simulink model "ASM_Traffic_V2X_Complete_Model_2"  (R2019a)
settings: Solver=ode1  StartTime=SIM.tstart.v  StopTime=Inf  FixedStep=SIM.StepSize.v  RelTol=1e-3
PostLoadFcn:
  | if any(exist('dsrtsu_mdlpostloadfcn', 'file') ~= 0), dsrtsu_mdlpostloadfcn('Execute', bdroot); end
  | try, asm_mdl_postloadfcn(bdroot, 'UpdateModel', 2200); catch, disp(lasterr); end,
undefined symbols (not defined in the file): _SensorPnts_1, _SensorPnts_13, _SensorPnts_17, _SensorPnts_21, _SensorPnts_25, _SensorPnts_29, _SensorPnts_33, _SensorPnts_37, _SensorPnts_41, _SensorPnts_45, _SensorPnts_49, _SensorPnts_5, _SensorPnts_53, _SensorPnts_57, _SensorPnts_9, _to_, CPT, G5A, ITS, MDL, rad, s_to_rpm, SIM
libraries: simulink x169, ASM_VehicleDynamics_lib x126, ASM_Traffic_lib x83, ASM_Utils_lib x49, mdbs x45, ASM_Environment_lib x17, dspindex x12, dsaV2xLibraryAux x10, dsmpblib x6, dsaV2xAsn1Library x4, dsaV2xLibrary x4, ASM_BrakeHydraulics_lib x4
(part 19 of 36)

== system ASM_Traffic_V2X_Complete_Model_2/MDL/Drivetrain/Transmission/AutomaticTransmission/ASMSignalCollector ==
  BusCreator : BusCreator  Inputs=3
  Signal Conversion : SignalConversion  OverrideOpt=off
  ASMSignalBus : Outport
  wires:
  [ASMBUS_Drivetrain_AutomaticTransmission_TorqueConverter] -> BusCreator/3
  BusCreator/1 -> Signal Conversion/1
  [ASMBUS_Drivetrain_AutomaticTransmission_Gearbox] -> BusCreator/2
  [ASMBUS_Drivetrain_AutomaticTransmission_LockUpClutch] -> BusCreator/1
  Signal Conversion/1 -> ASMSignalBus/1  "AutomaticTransmission"

== system ASM_Traffic_V2X_Complete_Model_2/MDL/Drivetrain/Transmission/AutomaticTransmission/Torque_Summation ==
  Trq_Fric[Nm] : Inport
  Trq_Out_LockupClutch[Nm] : Inport  Port=2
  Trq_Pump[Nm] : Inport  Port=3
  Trq_Turbine[Nm] : Inport  Port=4
  Sum1 : Sum  Inputs=2  SaturateOnIntegerOverflow=on  InputSameDT=on  OutDataTypeStr=Inherit: Same as first input
  Sum5 : Sum  Inputs=2  SaturateOnIntegerOverflow=on  InputSameDT=on  OutDataTypeStr=Inherit: Same as first input
  Trq_In_Converter[Nm] : Outport  InitialOutput=0
  Trq_In_Trm[Nm] : Outport  Port=2
  wires:
  Trq_Pump[Nm]/1 -> Sum5/1
  Sum1/1 -> Trq_In_Trm[Nm]/1
  Sum5/1 -> Trq_In_Converter[Nm]/1
  Trq_Fric[Nm]/1 -> Sum5/2
  Trq_Out_LockupClutch[Nm]/1 -> Sum1/1
  Trq_Turbine[Nm]/1 -> Sum1/2

== system ASM_Traffic_V2X_Complete_Model_2/MDL/Drivetrain/Transmission/ManualTransmission/ASMSignalCollector ==
  BusCreator : BusCreator  Inputs=2
  Signal Conversion : SignalConversion  OverrideOpt=off
  ASMSignalBus : Outport
  wires:
  BusCreator/1 -> Signal Conversion/1
  [ASMBUS_Drivetrain_ManualTransmission_Gearbox] -> BusCreator/2
  [ASMBUS_Drivetrain_ManualTransmission_Clutch] -> BusCreator/1
  Signal Conversion/1 -> ASMSignalBus/1  "ManualTransmission"

== system ASM_Traffic_V2X_Complete_Model_2/MDL/Environment/Driver/LateralController/ASMSignalCollector ==
  s_Preview_LatCtrl[m] : Inport
  Angle_SteeringWheel_LatCtrl[deg] : Inport  Port=2
  e_Lat[m] : Inport  Port=3
  Bus Creator : BusCreator  Inputs=3
  Bus Creator1 : BusCreator  Inputs=4
  Max : MinMax  Function=max  SaturateOnIntegerOverflow=on  InputSameDT=on
  tag scope: ASMBUS_Env_Driver_LatController=global
  wires:
  [ASMBUS_Env_Driver_LatCtrl_PosError] -> Bus Creator1/4
  Max/1 -> Bus Creator/1  "s_Preview_LatCtrl[m]"
  Angle_SteeringWheel_LatCtrl[deg]/1 -> Bus Creator/2  "Angle_SteeringWheel_LatCtrl[deg]"
  Bus Creator1/1 -> [ASMBUS_Env_Driver_LatController]  "LateralController"
  [ASMBUS_Env_Driver_LatCtrl2] -> Bus Creator1/3
  [ASMBUS_Env_Driver_LatCtrl1] -> Bus Creator1/2
  Bus Creator/1 -> Bus Creator1/1  "ActiveLateralController"
  e_Lat[m]/1 -> Bus Creator/3  "e_Lat[m]"
  s_Preview_LatCtrl[m]/1 -> Max/1  "s_Preview_LatCtrl[m]"

== system ASM_Traffic_V2X_Complete_Model_2/MDL/Environment/Driver/LongitudinalController/ASMSignalCollector ==
  Bus Creator : BusCreator  Inputs=2
  tag scope: ASMBUS_Env_Driver_LongController=global
  wires:
  [ASMBUS_Env_Driver_GearShifter] -> Bus Creator/2
  [ASMBUS_Env_Driver_LongCtrl] -> Bus Creator/1
  Bus Creator/1 -> [ASMBUS_Env_Driver_LongController]  "LongitudinalController"

== system ASM_Traffic_V2X_Complete_Model_2/MDL/Environment/Driver/LongitudinalController/Default_GearClutch_Mode ==
  note: For automatic transmission, the default value of GearClutch_Mode is set to the Driver Mode
  GearClutch_Mode[1Stim|2Driver|3OpenClutch|4RefGear] : Inport
  Automatic_Transmission : simulink/Logic and Bit Operations/Compare To Constant  relop===  const=2  OutDataTypeStr=boolean
  GearClutch_Mode[2Driver] : Constant  Value=2
  Multiport Switch : MultiPortSwitch  Inputs=2
  Sw_GearClutchMode[1Driver|2Others] : Constant
  Switch : Switch  Criteria=u2 ~= 0
  GearClutch_Mode[1Stim|2Driver|3OpenClutch|4RefGear]_ : Outport  OutputWhenDisabled=reset  InitialOutput=0
  wires:
  Multiport Switch/1 -> Switch/1
  Sw_GearClutchMode[1Driver|2Others]/1 -> Multiport Switch/1
  GearClutch_Mode[2Driver]/1 -> Multiport Switch/2
  GearClutch_Mode[1Stim|2Driver|3OpenClutch|4RefGear]/1 -> Multiport Switch/3, Switch/3
  Switch/1 -> GearClutch_Mode[1Stim|2Driver|3OpenClutch|4RefGear]_/1
  Automatic_Transmission/1 -> Switch/2
  [TAG_Sw_Transmission_Mode] -> Automatic_Transmission/1

== system ASM_Traffic_V2X_Complete_Model_2/MDL/Environment/Driver/LongitudinalController/Driving_Resistances ==
  VehicleDynamics_Signals : Inport
  Add : Sum  Inputs=+++
  Bus Selector1 : BusSelector  OutputSignals=VehicleMovement.Forces.F_x_Vehicle_Gravitational[N],VehicleMovement.Forces.F_x_Aero_CoorSys_V[N],VehicleMovement.Forces.F_z_Vehicle_Gravitational[N],Tire.Coef_RollingRes_Mean[]
  Gain : Gain  Gain=-1
  Gain1 : Gain
  Gain2 : Gain
  Product2 : Product  RndMeth=Zero
  F_Tractive_Res[N] : Outport
  wires:
  Gain1/1 -> Add/2  "F_Slope[N]"
  Gain2/1 -> Add/1  "F_Aerodynamics[N]"
  Bus Selector1/3 -> Product2/1  "<F_z_Vehicle_Gravitational[N]>"
  Bus Selector1/2 -> Gain1/1  "<F_x_Aero_CoorSys_V[N]>"
  Bus Selector1/1 -> Gain2/1  "<F_x_Vehicle_Gravitational[N]>"
  Gain/1 -> F_Tractive_Res[N]/1
  Add/1 -> Gain/1  "Driving_Res[N]"
  Product2/1 -> Add/3  "F_Roll[N]"
  Bus Selector1/4 -> Product2/2  "<Coef_RollingRes_Mean[]>"
  VehicleDynamics_Signals/1 -> Bus Selector1/1

== system ASM_Traffic_V2X_Complete_Model_2/MDL/Environment/Driver/ReferenceVelocity/Extend_Dimension ==
  In : Inport
  Selector : Selector  InputPortWidth=10  IndexOptions=Index vector (dialog)  Indices=[1:10,10,10,10,10,10]  OutputSizes=1
      settings: AttributesFormatString=|
      | PortWidth = %<InputPortWidth>
      | Indices = %<Indices>
  Out : Outport
  wires:
  In/1 -> Selector/1
  Selector/1 -> Out/1

== system ASM_Traffic_V2X_Complete_Model_2/MDL/Environment/Driver/ReferenceVelocity/Reduce_Dimension2 ==
  In : Inport
  Selector : Selector  InputPortWidth=15  IndexOptions=Index vector (dialog)  Indices=[1:10]  OutputSizes=1
      settings: AttributesFormatString=|
      | PortWidth = %<InputPortWidth>
      | Indices = %<Indices>
  Out : Outport
  wires:
  Selector/1 -> Out/1
  In/1 -> Selector/1

== system ASM_Traffic_V2X_Complete_Model_2/MDL/Environment/Driver/ReferenceVelocity/Reduce_Dimension3 ==
  In : Inport
  Selector : Selector  InputPortWidth=15  IndexOptions=Index vector (dialog)  Indices=[1:10]  OutputSizes=1
      settings: AttributesFormatString=|
      | PortWidth = %<InputPortWidth>
      | Indices = %<Indices>
  Out : Outport
  wires:
  In/1 -> Selector/1
  Selector/1 -> Out/1

== system ASM_Traffic_V2X_Complete_Model_2/MDL/Environment/Driver/ReferenceVelocity/Reduce_Dimension4 ==
  In : Inport
  Selector : Selector  InputPortWidth=15  IndexOptions=Index vector (dialog)  Indices=[1:10]  OutputSizes=1
      settings: AttributesFormatString=|
      | PortWidth = %<InputPortWidth>
      | Indices = %<Indices>
  Out : Outport
  wires:
  Selector/1 -> Out/1
  In/1 -> Selector/1

== system ASM_Traffic_V2X_Complete_Model_2/MDL/Environment/Driver/ReferenceVelocity/Reduce_Dimension5 ==
  In : Inport
  Selector : Selector  InputPortWidth=15  IndexOptions=Index vector (dialog)  Indices=[1:10]  OutputSizes=1
      settings: AttributesFormatString=|
      | PortWidth = %<InputPortWidth>
      | Indices = %<Indices>
  Out : Outport
  wires:
  Selector/1 -> Out/1
  In/1 -> Selector/1

== system ASM_Traffic_V2X_Complete_Model_2/MDL/Environment/Driver/SignalSelection/ASMSignalCollector ==
  Driver_Signals : Inport
  tag scope: ASMBUS_Env_Driver_SignalSelection=global
  wires:
  Driver_Signals/1 -> [ASMBUS_Env_Driver_SignalSelection]  "OutputSignals"

== system ASM_Traffic_V2X_Complete_Model_2/MDL/Environment/Driver/Source_of_eGoCAR_Control_Conditions/Steer_Decision_Conditions ==
  In1 : Inport
  AND : Logic  IconShape=distinctive  AllPortsSameDT=off  OutDataTypeStr=boolean
  Clock : Clock
  Data Type Conversion : DataTypeConversion  OutDataTypeStr=double
  Min_Speed_for_Manueveur : Constant  Value=50
  Min_Time_for_Manueveur : Constant  Value=10
  Relational Operator : RelationalOperator  OutDataTypeStr=boolean  RndMeth=Simplest
  Relational Operator1 : RelationalOperator  Operator=<=  OutDataTypeStr=boolean  RndMeth=Simplest
  Out1 : Outport
  wires:
  Relational Operator1/1 -> AND/2
  AND/1 -> Data Type Conversion/1
  Relational Operator/1 -> AND/1
  Min_Speed_for_Manueveur/1 -> Relational Operator1/2
  In1/1 -> Relational Operator1/1
  Clock/1 -> Relational Operator/1
  Min_Time_for_Manueveur/1 -> Relational Operator/2
  Data Type Conversion/1 -> Out1/1

== system ASM_Traffic_V2X_Complete_Model_2/MDL/Environment/EnvironmentInterface_In/Drivetrain/Mapping ==
  n_Engine[rpm]_ : Inport
  omega_Out_Trm[rad|s]_ : Inport  Port=2
  Bus Creator : BusCreator  Inputs=2
  n_Engine[rpm] : Subsystem
      mask Display: disp('')
  omega_Out_Trm[rad|s] : Subsystem
      mask Display: disp('')
  Out : Outport
  wires:
  omega_Out_Trm[rad|s]/1(Out1) -> Bus Creator/2  "omega_Out_Trm[rad|s]"
  n_Engine[rpm]/1(Out1) -> Bus Creator/1  "n_Engine[rpm]"
  omega_Out_Trm[rad|s]_/1 -> omega_Out_Trm[rad|s]/1(In1)
  n_Engine[rpm]_/1 -> n_Engine[rpm]/1(In1)
  Bus Creator/1 -> Out/1  "Drivetrain"

== system ASM_Traffic_V2X_Complete_Model_2/MDL/Environment/EnvironmentInterface_In/SoftECU_Engine/Mapping ==
  Const_n_Engine_Idle_Set[rpm] : Inport
  State_Engine[0|1|2|3|4] : Inport  Port=2
  FCW[0Off|1On] : Inport  Port=3
  AEB[0Off|1On] : Inport  Port=4
  AEB[0Off|1On]1 : Subsystem
      mask Display: disp('')
  Bus Creator : BusCreator  Inputs=2
  Bus Creator1 : BusCreator  Inputs=2
  Bus Creator2 : BusCreator  Inputs=2
  Const_n_Engine_Idle_Set[rpm]1 : Subsystem
      mask Display: disp('')
  FCW[0Off|1On]1 : Subsystem
      mask Display: disp('')
  State_Engine[0|1|2|3|4]_ : Subsystem
      mask Display: disp('')
  Out : Outport
  wires:
  State_Engine[0|1|2|3|4]_/1(Out1) -> Bus Creator/2  "State_Engine[0|1|2|3|4]"
  State_Engine[0|1|2|3|4]/1 -> State_Engine[0|1|2|3|4]_/1(In1)
  Bus Creator2/1 -> Out/1  "SoftECU"
  Bus Creator1/1 -> Bus Creator2/2  "SoftECU_ACC"
  Bus Creator/1 -> Bus Creator2/1  "SoftECU_Engine"
  AEB[0Off|1On]1/1(Out1) -> Bus Creator1/2  "AEB[0Off|1On]"
  FCW[0Off|1On]1/1(Out1) -> Bus Creator1/1  "FCW[0Off|1On]"
  AEB[0Off|1On]/1 -> AEB[0Off|1On]1/1(In1)
  FCW[0Off|1On]/1 -> FCW[0Off|1On]1/1(In1)
  Const_n_Engine_Idle_Set[rpm]1/1(Out1) -> Bus Creator/1  "Const_n_Engine_Idle_Set[rpm]"
  Const_n_Engine_Idle_Set[rpm]/1 -> Const_n_Engine_Idle_Set[rpm]1/1(In1)

== system ASM_Traffic_V2X_Complete_Model_2/MDL/Environment/EnvironmentInterface_In/Steering/Mapping ==
  i_Steering_Mean[] : Inport
  Angle_SteeringWheel[deg] : Inport  Port=2
  Trq_SteeringWheel[Nm] : Inport  Port=3
  Angle_SteeringWheel[deg]1 : Subsystem
      mask Display: disp('')
  Bus Creator : BusCreator  Inputs=3
  Trq_SteeringWheel[Nm]1 : Subsystem
      mask Display: disp('')
  i_Steering_Mean[]1 : Subsystem
      mask Display: disp('')
  Out : Outport
  wires:
  Angle_SteeringWheel[deg]1/1(Out1) -> Bus Creator/2  "Angle_SteeringWheel[deg]"
  Trq_SteeringWheel[Nm]1/1(Out1) -> Bus Creator/3  "Trq_SteeringWheel[Nm]"
  Angle_SteeringWheel[deg]/1 -> Angle_SteeringWheel[deg]1/1(In1)
  Trq_SteeringWheel[Nm]/1 -> Trq_SteeringWheel[Nm]1/1(In1)
  i_Steering_Mean[]/1 -> i_Steering_Mean[]1/1(In1)
  i_Steering_Mean[]1/1(Out1) -> Bus Creator/1  "i_Steering_Mean[]"
  Bus Creator/1 -> Out/1  "Steering"

== system ASM_Traffic_V2X_Complete_Model_2/MDL/Environment/EnvironmentInterface_In/Tire/Mapping ==
  r_Dyn_Tire_Mean[m] : Inport
  Coef_RollingRes_Mean[] : Inport  Port=2
  CorneringStiffness_Tire_Front[N|rad] : Inport  Port=3
  CorneringStiffness_Tire_Rear[N|rad] : Inport  Port=4
  Pos_CP_FL_CoorSys_E[x;y][m] : Inport  Port=5
  Pos_CP_FR_CoorSys_E[x;y][m] : Inport  Port=6
  Pos_CP_RL_CoorSys_E[x;y][m] : Inport  Port=7
  Pos_CP_RR_CoorSys_E[x;y][m] : Inport  Port=8
  Bus Creator : BusCreator  Inputs=5
  Coef_RollingRes_Mean[]1 : Subsystem
      mask Display: disp('')
  CorneringStiffness_Tire_Front[N|rad]1 : Subsystem
      mask Display: disp('')
  CorneringStiffness_Tire_Rear[N|rad]1 : Subsystem
      mask Display: disp('')
  Mux : Mux
  r_Dyn_Tire_Mean[m]1 : Subsystem
      mask Display: disp('')
  Out : Outport
  wires:
  Mux/1 -> Bus Creator/5  "Pos_CP_CoorSys_E[:][x;y][m]"
  CorneringStiffness_Tire_Rear[N|rad]/1 -> CorneringStiffness_Tire_Rear[N|rad]1/1(In1)
  CorneringStiffness_Tire_Front[N|rad]/1 -> CorneringStiffness_Tire_Front[N|rad]1/1(In1)
  Coef_RollingRes_Mean[]/1 -> Coef_RollingRes_Mean[]1/1(In1)
  r_Dyn_Tire_Mean[m]/1 -> r_Dyn_Tire_Mean[m]1/1(In1)
  CorneringStiffness_Tire_Rear[N|rad]1/1(Out1) -> Bus Creator/4  "CorneringStiffness_Tire_Rear[N|rad]"
  CorneringStiffness_Tire_Front[N|rad]1/1(Out1) -> Bus Creator/3  "CorneringStiffness_Tire_Front[N|rad]"
  Coef_RollingRes_Mean[]1/1(Out1) -> Bus Creator/2  "Coef_RollingRes_Mean[]"
  r_Dyn_Tire_Mean[m]1/1(Out1) -> Bus Creator/1  "r_Dyn_Tire_Mean[m]"
  Pos_CP_RR_CoorSys_E[x;y][m]/1 -> Mux/4
  Pos_CP_RL_CoorSys_E[x;y][m]/1 -> Mux/3
  Pos_CP_FR_CoorSys_E[x;y][m]/1 -> Mux/2
  Pos_CP_FL_CoorSys_E[x;y][m]/1 -> Mux/1
  Bus Creator/1 -> Out/1  "Tire"

== system ASM_Traffic_V2X_Complete_Model_2/MDL/Environment/EnvironmentInterface_In/VehicleMovement/Mapping ==
  m_TotalVehicle[kg] : Inport
  Pos_x_CoG_Vehicle_Total[m] : Inport  Port=2
  Inertia_z_Vehicle_Total[kgm2] : Inport  Port=3
  Bus Creator : BusCreator  Inputs=3
  Inertia_z_Vehicle_Total[kgm2]1 : Subsystem
      mask Display: disp('')
  Pos_x_CoG_Vehicle_Total[m]1 : Subsystem
      mask Display: disp('')
  m_TotalVehicle[kg]1 : Subsystem
      mask Display: disp('')
  Out : Outport
  wires:
  Bus Creator/1 -> Out/1  "Parameters"
  m_TotalVehicle[kg]1/1(Out1) -> Bus Creator/1  "m_TotalVehicle[kg]"
  Pos_x_CoG_Vehicle_Total[m]1/1(Out1) -> Bus Creator/2  "Pos_x_CoG_Vehicle_Total[m]"
  Inertia_z_Vehicle_Total[kgm2]1/1(Out1) -> Bus Creator/3  "Inertia_z_Vehicle_Total[kgm2]"
  m_TotalVehicle[kg]/1 -> m_TotalVehicle[kg]1/1(In1)
  Pos_x_CoG_Vehicle_Total[m]/1 -> Pos_x_CoG_Vehicle_Total[m]1/1(In1)
  Inertia_z_Vehicle_Total[kgm2]/1 -> Inertia_z_Vehicle_Total[kgm2]1/1(In1)

== system ASM_Traffic_V2X_Complete_Model_2/MDL/Environment/EnvironmentInterface_In/VehicleMovement/Mapping_Acc ==
  a_y_Vehicle_CoG[m|s2] : Inport
  Bus Creator : BusCreator  Inputs=1
  a_y_Vehicle_CoG[m|s2]1 : Subsystem
      mask Display: disp('')
  Out : Outport
  wires:
  Bus Creator/1 -> Out/1  "Accelerations"
  a_y_Vehicle_CoG[m|s2]1/1(Out1) -> Bus Creator/1  "a_y_Vehicle_CoG[m|s2]"
  a_y_Vehicle_CoG[m|s2]/1 -> a_y_Vehicle_CoG[m|s2]1/1(In1)

== system ASM_Traffic_V2X_Complete_Model_2/MDL/Environment/EnvironmentInterface_In/VehicleMovement/Mapping_F ==
  F_x_Vehicle_Gravitational[N] : Inport
  F_z_Vehicle_Gravitational[N] : Inport  Port=2
  F_x_Aero_CoorSys_V[N] : Inport  Port=3
  Bus Creator : BusCreator  Inputs=3
  F_x_Aero_CoorSys_V[N]1 : Subsystem
      mask Display: disp('')
  F_x_Vehicle_Gravitational[N]1 : Subsystem
      mask Display: disp('')
  F_z_Vehicle_Gravitational[N]1 : Subsystem
      mask Display: disp('')
  Out : Outport
  wires:
  F_x_Aero_CoorSys_V[N]1/1(Out1) -> Bus Creator/3  "F_x_Aero_CoorSys_V[N]"
  F_x_Aero_CoorSys_V[N]/1 -> F_x_Aero_CoorSys_V[N]1/1(In1)
  F_z_Vehicle_Gravitational[N]/1 -> F_z_Vehicle_Gravitational[N]1/1(In1)
  F_x_Vehicle_Gravitational[N]/1 -> F_x_Vehicle_Gravitational[N]1/1(In1)
  F_z_Vehicle_Gravitational[N]1/1(Out1) -> Bus Creator/2  "F_z_Vehicle_Gravitational[N]"
  Bus Creator/1 -> Out/1  "Forces"
  F_x_Vehicle_Gravitational[N]1/1(Out1) -> Bus Creator/1  "F_x_Vehicle_Gravitational[N]"

== system ASM_Traffic_V2X_Complete_Model_2/MDL/Environment/EnvironmentInterface_In/VehicleMovement/Mapping_Pos ==
  Pos_Vehicle_CoorSys_E[x;y;z][m] : Inport
  Angle_Vehicle_CoorSys_E[x;y;z][deg] : Inport  Port=2
  s_Vehicle[m] : Inport  Port=3
  RotationMatrix_V_to_E[3x3] : Inport  Port=4
  Bus Creator : BusCreator  Inputs=4
  Bus Creator1 : BusCreator  Inputs=4
  Bus Creator2 : BusCreator  Inputs=4
  Bus Selector : BusSelector  OutputSignals=Pos_x_Vehicle_CoorSys_E[m],Pos_y_Vehicle_CoorSys_E[m],Pos_z_Vehicle_CoorSys_E[m]
  Bus Selector1 : BusSelector  OutputSignals=Angle_Roll_Vehicle_CoorSys_E[deg],Angle_Pitch_Vehicle_CoorSys_E[deg],Angle_Yaw_Vehicle_CoorSys_E[deg]
  Demux : Demux  Outputs=3
  Demux1 : Demux  Outputs=3
  Mux : Mux  Inputs=3
  Mux1 : Mux  Inputs=3
  RotationMatrix_V_to_E[3x3]1 : Subsystem
      mask Display: disp('')
  SignalSpec_Dim3_1 : SignalSpecification  Dimensions=3
  SignalSpec_Dim3_2 : SignalSpecification  Dimensions=3
  s_Vehicle[m]1 : Subsystem
      mask Display: disp('')
  Out : Outport
  wires:
  RotationMatrix_V_to_E[3x3]1/1(Out1) -> Bus Creator/4  "RotationMatrix_V_to_E[3x3]"
  RotationMatrix_V_to_E[3x3]/1 -> RotationMatrix_V_to_E[3x3]1/1(In1)
  Bus Creator/1 -> Out/1  "Positions"
  Bus Creator1/1 -> Bus Creator/1  "Pos_Vehicle_CoorSys_E[x;y;z][m]"
  Bus Creator2/1 -> Bus Creator/2  "Angle_Vehicle_CoorSys_E[x;y;z][deg]"
  s_Vehicle[m]1/1(Out1) -> Bus Creator/3  "s_Vehicle[m]"
  s_Vehicle[m]/1 -> s_Vehicle[m]1/1(In1)
  SignalSpec_Dim3_1/1 -> Bus Creator1/4, Demux/1  "Pos_Vehicle_CoorSys_E[x;y;z][m]"
  SignalSpec_Dim3_2/1 -> Bus Creator2/4, Demux1/1  "Angle_Vehicle_CoorSys_E[x;y;z][deg]"
  Demux/1 -> Bus Creator1/1  "Pos_x_Vehicle_CoorSys_E[m]"
  Demux/2 -> Bus Creator1/2  "Pos_y_Vehicle_CoorSys_E[m]"
  Demux/3 -> Bus Creator1/3  "Pos_z_Vehicle_CoorSys_E[m]"
  Demux1/3 -> Bus Creator2/3  "Angle_Yaw_Vehicle_CoorSys_E[deg]"
  Demux1/1 -> Bus Creator2/1  "Angle_Roll_Vehicle_CoorSys_E[deg]"
  Demux1/2 -> Bus Creator2/2  "Angle_Pitch_Vehicle_CoorSys_E[deg]"
  Pos_Vehicle_CoorSys_E[x;y;z][m]/1 -> Bus Selector/1
  Bus Selector/2 -> Mux/2  "<Pos_y_Vehicle_CoorSys_E[m]>"
  Bus Selector/1 -> Mux/1  "<Pos_x_Vehicle_CoorSys_E[m]>"
  Bus Selector/3 -> Mux/3  "<Pos_z_Vehicle_CoorSys_E[m]>"
  Mux/1 -> SignalSpec_Dim3_1/1
  Angle_Vehicle_CoorSys_E[x;y;z][deg]/1 -> Bus Selector1/1
  Bus Selector1/2 -> Mux1/2  "<Angle_Pitch_Vehicle_CoorSys_E[deg]>"
  Bus Selector1/1 -> Mux1/1  "<Angle_Roll_Vehicle_CoorSys_E[deg]>"
  Bus Selector1/3 -> Mux1/3  "<Angle_Yaw_Vehicle_CoorSys_E[deg]>"
  Mux1/1 -> SignalSpec_Dim3_2/1

== system ASM_Traffic_V2X_Complete_Model_2/MDL/Environment/EnvironmentInterface_In/VehicleMovement/Mapping_Vel ==
  v_x_Vehicle_CoG[km|h] : Inport
  v_y_Vehicle_CoG[km|h] : Inport  Port=2
  RollRate_Vehicle_CoG[deg|s] : Inport  Port=3
  YawRate_Vehicle_CoG[deg|s] : Inport  Port=4
  Bus Creator : BusCreator  Inputs=4
  RollRate_Vehicle_CoG[deg|s]1 : Subsystem
      mask Display: disp('')
  YawRate_Vehicle_CoG[deg|s]1 : Subsystem
      mask Display: disp('')
  v_x_Vehicle_CoG[km|h]1 : Subsystem
      mask Display: disp('')
  v_y_Vehicle_CoG[km|h]1 : Subsystem
      mask Display: disp('')
  Out : Outport
  wires:
  Bus Creator/1 -> Out/1  "Velocities"
  v_x_Vehicle_CoG[km|h]1/1(Out1) -> Bus Creator/1  "v_x_Vehicle[km|h]"
  v_y_Vehicle_CoG[km|h]1/1(Out1) -> Bus Creator/2  "v_y_Vehicle[km|h]"
  RollRate_Vehicle_CoG[deg|s]1/1(Out1) -> Bus Creator/3  "RollRate_Vehicle[deg|s]"
  YawRate_Vehicle_CoG[deg|s]1/1(Out1) -> Bus Creator/4  "YawRate_Vehicle[deg|s]"
  v_x_Vehicle_CoG[km|h]/1 -> v_x_Vehicle_CoG[km|h]1/1(In1)
  v_y_Vehicle_CoG[km|h]/1 -> v_y_Vehicle_CoG[km|h]1/1(In1)
  RollRate_Vehicle_CoG[deg|s]/1 -> RollRate_Vehicle_CoG[deg|s]1/1(In1)
  YawRate_Vehicle_CoG[deg|s]/1 -> YawRate_Vehicle_CoG[deg|s]1/1(In1)

== system ASM_Traffic_V2X_Complete_Model_2/MDL/Environment/Maneuver/Customize_UserSignals/CustomizedUserSignals ==
  User1[] : Inport
  User2[] : Inport  Port=2
  User3[] : Inport  Port=3
  User4[] : Inport  Port=4
  User5[] : Inport  Port=5
  User6[] : Inport  Port=6
  User7[] : Inport  Port=7
  User8[] : Inport  Port=8
  Gain{1..8} (8 alike) : Gain
  ExternalSegmentEnd_Mode[] : Outport
  ExternalSegmentEnd_Value[] : Outport  Port=2
  ASM_Vehicle_TurnLights[] : Outport  Port=3
  ECU_Commands[] : Outport  Port=4
  Mnv_DataStream_5[] : Outport  Port=5
  Mnv_DataStream_6[] : Outport  Port=6
  Mnv_DataStream_7[] : Outport  Port=7
  Mnv_DataStream_8[] : Outport  Port=8
  wires:
  Gain8/1 -> Mnv_DataStream_8[]/1  "Mnv_DataStream_8[]"
  Gain7/1 -> Mnv_DataStream_7[]/1  "Mnv_DataStream_7[]"
  Gain6/1 -> Mnv_DataStream_6[]/1  "Mnv_DataStream_6[]"
  Gain5/1 -> Mnv_DataStream_5[]/1  "Mnv_DataStream_5[]"
  User8[]/1 -> Gain8/1
  User7[]/1 -> Gain7/1
  User6[]/1 -> Gain6/1
  User5[]/1 -> Gain5/1
  Gain3/1 -> ASM_Vehicle_TurnLights[]/1  "ASM_Vehicle_TurnLights[]"
  User3[]/1 -> Gain3/1
  User2[]/1 -> Gain2/1
  User1[]/1 -> Gain1/1
  Gain4/1 -> ECU_Commands[]/1  "ECU_Commands[]"
  User4[]/1 -> Gain4/1
  Gain2/1 -> ExternalSegmentEnd_Value[]/1  "ExternalSegmentEnd_Value[]"
  Gain1/1 -> ExternalSegmentEnd_Mode[]/1  "ExternalSegmentEnd_Mode[]"

== system ASM_Traffic_V2X_Complete_Model_2/MDL/Environment/Maneuver/ExternalSegmentEnd/Dist_Front_Min ==
  Dist_Front[m] : Inport
  Min : MinMax
  Replace_NoObjectFound1 : Subsystem
      mask Display: disp ('<= 0 --> 1000')
  Out1 : Outport
  wires:
  Dist_Front[m]/1 -> Replace_NoObjectFound1/1(In1)
  Min/1 -> Out1/1
  Replace_NoObjectFound1/1(Out1) -> Min/1

== system ASM_Traffic_V2X_Complete_Model_2/MDL/Environment/Maneuver/ExternalSegmentEnd/Dist_Rear_Min ==
  Dist_Rear[m] : Inport
  Min : MinMax
  Replace_NoObjectFound1 : Subsystem
      mask Display: disp ('<= 0 --> 1000')
  Out1 : Outport
  wires:
  Replace_NoObjectFound1/1(Out1) -> Min/1
  Min/1 -> Out1/1
  Dist_Rear[m]/1 -> Replace_NoObjectFound1/1(In1)

== system ASM_Traffic_V2X_Complete_Model_2/MDL/Environment/Maneuver/ExternalSegmentEnd/SegmentEndTrigger ==
  ExternalSegmentEnd_Mode[] : Inport
  ExternalSegmentEnd_Value[] : Inport  Port=2
  s_Road[m] : Inport  Port=3
  RollRate_Vehicle[deg|s] : Inport  Port=4
  Distance_Front[m] : Inport  Port=5
  Distance_Rear[m] : Inport  Port=6
  Const_0 : Constant  Value=0
  Const_Nr_SegEndModes_Max[] : Constant  Value=4
  Fishhook : Subsystem
  Multiport Switch : MultiPortSwitch  DataPortOrder=Zero-based contiguous  Inputs=5  zeroidx=on
  RelOp_DistFrontSmaller : RelationalOperator  Operator=<=  OutDataTypeStr=boolean  RndMeth=Nearest
  RelOp_DistRearSmaller : RelationalOperator  Operator=<=  OutDataTypeStr=boolean  RndMeth=Nearest
  RelOp_PosBigger : RelationalOperator  OutDataTypeStr=boolean  RndMeth=Nearest
  SaturateAndRound : Subsystem
  External_SegmentEnd[0|1] : Outport
  wires:
  Multiport Switch/1 -> External_SegmentEnd[0|1]/1
  RelOp_PosBigger/1 -> Multiport Switch/3
  Const_0/1 -> Multiport Switch/2
  ExternalSegmentEnd_Value[]/1 -> RelOp_PosBigger/2, Fishhook/1(RollRate_Threshold[deg|s]), RelOp_DistFrontSmaller/2, RelOp_DistRearSmaller/2
  s_Road[m]/1 -> RelOp_PosBigger/1
  RollRate_Vehicle[deg|s]/1 -> Fishhook/2(RollRate_Vehicle_CoG[deg|s])
  Fishhook/1(SegmentEnd_Fishhook) -> Multiport Switch/4
  Const_Nr_SegEndModes_Max[]/1 -> SaturateAndRound/2(Max)
  ExternalSegmentEnd_Mode[]/1 -> SaturateAndRound/1(In)
  SaturateAndRound/1(ExternalSegmentEnd_Mode[]) -> Multiport Switch/1
  Distance_Front[m]/1 -> RelOp_DistFrontSmaller/1
  Distance_Rear[m]/1 -> RelOp_DistRearSmaller/1
  RelOp_DistFrontSmaller/1 -> Multiport Switch/5
  RelOp_DistRearSmaller/1 -> Multiport Switch/6

== system ASM_Traffic_V2X_Complete_Model_2/MDL/Environment/Maneuver/ReplaceBrake/ReplaceEnable ==
  ManeuverState : Inport
  Sw_MasterBrakeCylinder_Mode[1linear|2physical] : Inport  Port=2
  Const_BrakeState : Constant  Value=4
  Const_WaitState : Constant  Value=5
  Const_physType : Constant  Value=2
  LogOpOr : Logic  Operator=OR  AllPortsSameDT=off  OutDataTypeStr=boolean
  Logical Operator : Logic  AllPortsSameDT=off  OutDataTypeStr=boolean
  RelOpBrake : RelationalOperator  Operator===  OutDataTypeStr=boolean  RndMeth=Nearest
  RelOpConst_physType : RelationalOperator  Operator===  OutDataTypeStr=boolean  RndMeth=Nearest
  RelOpWait : RelationalOperator  Operator===  OutDataTypeStr=boolean  RndMeth=Nearest
  ReplaceEnable[0Off|1On] : Outport
  wires:
  LogOpOr/1 -> Logical Operator/1
  RelOpWait/1 -> LogOpOr/2
  RelOpBrake/1 -> LogOpOr/1
  Logical Operator/1 -> ReplaceEnable[0Off|1On]/1
  RelOpConst_physType/1 -> Logical Operator/2
  Const_physType/1 -> RelOpConst_physType/2
  Sw_MasterBrakeCylinder_Mode[1linear|2physical]/1 -> RelOpConst_physType/1
  Const_WaitState/1 -> RelOpWait/2
  Const_BrakeState/1 -> RelOpBrake/2
  ManeuverState/1 -> RelOpWait/1, RelOpBrake/1

== system ASM_Traffic_V2X_Complete_Model_2/MDL/Environment/Maneuver/Reset _IfModeSwitched/IgnoreSimulationStart ==
  Reset_In : Inport
  Constant : Constant
  Memory1 : Memory
  Product : Product  SaturateOnIntegerOverflow=on  OutDataTypeStr=Inherit: Same as first input
  Reset_Out : Outport
  wires:
  Constant/1 -> Memory1/1
  Memory1/1 -> Product/2
  Reset_In/1 -> Product/1
  Product/1 -> Reset_Out/1

== system ASM_Traffic_V2X_Complete_Model_2/MDL/Environment/Maneuver/SimulationControl/KeepVehiclePosition ==
  Angle_Roll_Vehicle_CoorSys_E[deg] : Inport
  Angle_Pitch_Vehicle_CoorSys_E[deg] : Inport  Port=2
  Abs : Abs
  Logical Operator : Logic  Operator=OR  Inputs=1  AllPortsSameDT=off  OutDataTypeStr=boolean
  Logical Operator1 : Logic  AllPortsSameDT=off
  Memory : Memory  InheritSampleTime=on
  Mux : Mux  Inputs=2
  Relational Operator : RelationalOperator  Operator=>  OutDataTypeStr=boolean  RndMeth=Nearest
  Keep_VehiclePosition[0|1] : Outport
  wires:
  Mux/1 -> Abs/1
  Abs/1 -> Relational Operator/1
  [Tag_MaxAngleRollPitch] -> Relational Operator/2
  Relational Operator/1 -> Logical Operator/1
  Logical Operator/1 -> Memory/1
  Memory/1 -> Logical Operator1/1
  [Tag_Sw_Keep_VehiclePosition] -> Logical Operator1/2
  Logical Operator1/1 -> Keep_VehiclePosition[0|1]/1
  Angle_Roll_Vehicle_CoorSys_E[deg]/1 -> Mux/1
  Angle_Pitch_Vehicle_CoorSys_E[deg]/1 -> Mux/2

== system ASM_Traffic_V2X_Complete_Model_2/MDL/Environment/Road/Customize_UserSignals/CustomizedUserSignals ==
  User1[] : Inport
  User2[] : Inport  Port=2
  User3[] : Inport  Port=3
  Gain1 : Gain
  Gain2 : Gain
  Gain3 : Gain
  GPS_Method[] : Outport
  Const_Offset_Lat[deg] : Outport  Port=2
  Const_Offset_Long[deg] : Outport  Port=3
  wires:
  User2[]/1 -> Gain2/1
  User1[]/1 -> Gain1/1
  User3[]/1 -> Gain3/1
  Gain3/1 -> Const_Offset_Long[deg]/1  "Const_Offset_Long[deg]"
  Gain2/1 -> Const_Offset_Lat[deg]/1  "Const_Offset_Lat[deg]"
  Gain1/1 -> GPS_Method[]/1  "GPS_Method[]"

== system ASM_Traffic_V2X_Complete_Model_2/MDL/Environment/Road/SignalRouting/Mapping_CP ==
  In1 : Inport
  Bus Creator3 : BusCreator  Inputs=4
  Bus Selector1 : BusSelector  OutputSignals=Pos_z_CP[:][m],Fric_Coeff_CP[:][],UnitVec_z_CP[:][x;y;z],Sw_Tire_Parameter_Set_CP[:][1|2|3|4]
  Signal Specification : SignalSpecification  Dimensions=4
  Signal Specification1 : SignalSpecification  Dimensions=12
  Signal Specification2 : SignalSpecification  Dimensions=4
  Signal Specification3 : SignalSpecification  Dimensions=4
  Out1 : Outport
  wires:
  Signal Specification/1 -> Bus Creator3/1  "Pos_z_CP[FL;FR;RL;RR][m]"
  Signal Specification3/1 -> Bus Creator3/4  "Sw_Tire_Parameter_Set_CP[FL;FR;RL;RR][1|2|3|4]"
  Signal Specification1/1 -> Bus Creator3/3  "UnitVec_z_CP[FL;FR;RL;RR][x;y;z]"
  Signal Specification2/1 -> Bus Creator3/2  "Fric_Coeff_CP[FL;FR;RL;RR][]"
  Bus Creator3/1 -> Out1/1  "Road_ContactPoints"
  In1/1 -> Bus Selector1/1
  Bus Selector1/1 -> Signal Specification/1  "<Pos_z_CP[:][m]>"
  Bus Selector1/2 -> Signal Specification2/1  "<Fric_Coeff_CP[:][]>"
  Bus Selector1/3 -> Signal Specification1/1  "<UnitVec_z_CP[:][x;y;z]>"
  Bus Selector1/4 -> Signal Specification3/1  "<Sw_Tire_Parameter_Set_CP[:][1|2|3|4]>"

== system ASM_Traffic_V2X_Complete_Model_2/MDL/Environment/Traffic/FellowMovement/ASMSignalBusCollect ==
  d_Total_Fellows_Road[m] : Inport
  LaneIdx_Total_Fellows_Road[] : Inport  Port=2
  s_Fellows_Road[m] : Inport  Port=3
  v_Fellows_In[km|h] : Inport  Port=4
  Bus Creator2 : BusCreator  Inputs=4
  ASMSignalBus : Outport
  wires:
  d_Total_Fellows_Road[m]/1 -> Bus Creator2/1  "d_Total_Fellows[m]"
  LaneIdx_Total_Fellows_Road[]/1 -> Bus Creator2/2  "LaneIdx_Total_Fellows[]"
  s_Fellows_Road[m]/1 -> Bus Creator2/3  "s_Fellows[m]"
  v_Fellows_In[km|h]/1 -> Bus Creator2/4  "v_Fellows[km|h]"
  Bus Creator2/1 -> ASMSignalBus/1  "FellowMovement"

== system ASM_Traffic_V2X_Complete_Model_2/MDL/Environment/Traffic/FellowMovement/ASMSignalCollector ==
  Bus Creator1 : BusCreator  Inputs=5
  tag scope: ASMBUS_Environment_Traffic_FellowMovement=global
  wires:
  [ASMBUS_Traffic_FellowVelocities] -> Bus Creator1/3
  [ASMBUS_Traffic_UserSignals_Customized] -> Bus Creator1/5
  [ASMBUS_Traffic_TrafficScheduler] -> Bus Creator1/4
  [ASMBUS_Traffic_FellowPositions] -> Bus Creator1/2
  [ASMBUS_Traffic_FellowSignalLabels] -> Bus Creator1/1
  Bus Creator1/1 -> [ASMBUS_Environment_Traffic_FellowMovement]  "FellowMovement"

== system ASM_Traffic_V2X_Complete_Model_2/MDL/Environment/Traffic/FellowMovement/Customize_UserSignals ==
  UserSignals_In : Inport
  UserSignalsFellow_In : Inport  Port=2
  Bus Creator1 : BusCreator  Inputs=16
  Bus Selector : BusSelector  OutputSignals=User2[]
  Bus Selector1 : BusSelector  OutputSignals=UserSignals_Fellow1[],UserSignals_Fellow2[],UserSignals_Fellow3[],UserSignals_Fellow4[],UserSignals_Fellow5[],UserSignals_Fellow6[],UserSignals_Fellow7[],UserSignals_Fellow8[],UserSignals_Fellow9[],UserSignals_Fellow10[],UserSignals_Fellow11[],UserSignals_Fellow12[],UserSignals_Fellow13[],UserSignals_Fellow14[],UserSignals_Fellow15[]
  Label : Subsystem
  Label1 : Subsystem
  Label10 : Subsystem
  Label11 : Subsystem
  Label12 : Subsystem
  Label13 : Subsystem
  Label14 : Subsystem
  Label2 : Subsystem
  Label3 : Subsystem
  Label4 : Subsystem
  Label5 : Subsystem
  Label6 : Subsystem
  Label7 : Subsystem
  Label8 : Subsystem
  Label9 : Subsystem
  Memory : Memory
  Saturation : Saturate  UpperLimit=1  LowerLimit=0
  Selector{,1..14} (15 alike) : Selector  InputPortWidth=MDL.Traffic.MaxNumFDUserSignals.v  IndexOptions=Index vector (dialog)  Indices=[1]  OutputSizes=1
  Sum : Sum  Inputs=|-+  SaturateOnIntegerOverflow=on
  ASMSignalBus : Outport
  UserSignals_Customized : Outport  Port=2
  wires:
  Bus Selector1/15 -> Selector14/1  "<UserSignals_Fellow15[]>"
  Bus Selector1/14 -> Selector13/1  "<UserSignals_Fellow14[]>"
  Bus Selector1/11 -> Selector10/1  "<UserSignals_Fellow11[]>"
  Bus Selector1/12 -> Selector11/1  "<UserSignals_Fellow12[]>"
  Bus Selector1/9 -> Selector8/1  "<UserSignals_Fellow9[]>"
  Bus Selector1/10 -> Selector9/1  "<UserSignals_Fellow10[]>"
  Bus Selector1/13 -> Selector12/1  "<UserSignals_Fellow13[]>"
  Bus Selector1/8 -> Selector7/1  "<UserSignals_Fellow8[]>"
  Bus Selector1/7 -> Selector6/1  "<UserSignals_Fellow7[]>"
  Bus Selector1/3 -> Selector2/1  "<UserSignals_Fellow3[]>"
  Bus Selector1/4 -> Selector3/1  "<UserSignals_Fellow4[]>"
  Bus Selector1/1 -> Selector/1  "<UserSignals_Fellow1[]>"
  Bus Selector1/5 -> Selector4/1  "<UserSignals_Fellow5[]>"
  Bus Selector1/6 -> Selector5/1  "<UserSignals_Fellow6[]>"
  Bus Selector1/2 -> Selector1/1  "<UserSignals_Fellow2[]>"
  Selector14/1 -> Label14/1(In1)
  Selector13/1 -> Label13/1(In1)
  Selector12/1 -> Label12/1(In1)
  Selector11/1 -> Label11/1(In1)
  Selector10/1 -> Label10/1(In1)
  Selector9/1 -> Label9/1(In1)
  Selector8/1 -> Label8/1(In1)
  Selector7/1 -> Label7/1(In1)
  Selector6/1 -> Label6/1(In1)
  Selector5/1 -> Label5/1(In1)
  Selector4/1 -> Label4/1(In1)
  Selector3/1 -> Label3/1(In1)
  Selector2/1 -> Label2/1(In1)
  Selector1/1 -> Label1/1(In1)
  UserSignalsFellow_In/1 -> Bus Selector1/1
  Label14/1(Out1) -> Bus Creator1/16  "Fellow15_TurnLights"
  Label11/1(Out1) -> Bus Creator1/13  "Fellow12_TurnLights"
  Label12/1(Out1) -> Bus Creator1/14  "Fellow13_TurnLights"
  Label13/1(Out1) -> Bus Creator1/15  "Fellow14_TurnLights"
  Label9/1(Out1) -> Bus Creator1/11  "Fellow10_TurnLights"
  Label10/1(Out1) -> Bus Creator1/12  "Fellow11_TurnLights"
  Label6/1(Out1) -> Bus Creator1/8  "Fellow7_TurnLights"
  Label7/1(Out1) -> Bus Creator1/9  "Fellow8_TurnLights"
  Label8/1(Out1) -> Bus Creator1/10  "Fellow9_TurnLights"
  Label3/1(Out1) -> Bus Creator1/5  "Fellow4_TurnLights"
  Label4/1(Out1) -> Bus Creator1/6  "Fellow5_TurnLights"
  Label5/1(Out1) -> Bus Creator1/7  "Fellow6_TurnLights"
  Bus Creator1/1 -> UserSignals_Customized/1, ASMSignalBus/1  "UserSignals_Customized"
  Saturation/1 -> Bus Creator1/1  "ManeuverSegmentEndTrigger[0|1]"
  UserSignals_In/1 -> Bus Selector/1  "UserSignals"
  Bus Selector/1 -> Memory/1, Sum/2  "<User2[]>"
  Sum/1 -> Saturation/1
  Memory/1 -> Sum/1
  Selector/1 -> Label/1(In1)
  Label/1(Out1) -> Bus Creator1/2  "Fellow1_TurnLights"
  Label1/1(Out1) -> Bus Creator1/3  "Fellow2_TurnLights"
  Label2/1(Out1) -> Bus Creator1/4  "Fellow3_TurnLights"

== system ASM_Traffic_V2X_Complete_Model_2/MDL/Environment/Traffic/FellowMovement/External_Route ==
  Const_RouteDirection_Fellows_External[] : Constant  Value=zeros(1,MDL.Traffic.MaxNumFellows.v)
  Const_RouteId_Fellows_External[] : Constant  Value=zeros(1,MDL.Traffic.MaxNumFellows.v)
  RouteId_External[] : Outport
  RouteDirection_External[1|-1] : Outport  Port=2
  wires:
  Const_RouteDirection_Fellows_External[]/1 -> RouteDirection_External[1|-1]/1
  Const_RouteId_Fellows_External[]/1 -> RouteId_External[]/1

== system ASM_Traffic_V2X_Complete_Model_2/MDL/Environment/Traffic/FellowMovement/External_Signals ==
  Const_LaneIdx_Fellows_External[] : Constant  Value=zeros(1,MDL.Traffic.MaxNumFellows.v)
  Const_d_Fellows_External[m] : Constant  Value=zeros(1,MDL.Traffic.MaxNumFellows.v)
  Const_s_Fellows_External[m] : Constant  Value=zeros(1,MDL.Traffic.MaxNumFellows.v)
  Const_tgap_Fellows_External[s] : Constant  Value=zeros(1,MDL.Traffic.MaxNumFellows.v)
  Const_v_Fellows_External[km|h] : Constant  Value=zeros(1,MDL.Traffic.MaxNumFellows.v)
  s_Fellows_External[m] : Outport
  v_Fellows_External[km|h] : Outport  Port=2
  d_Fellows_External[m] : Outport  Port=3
  tgap_Fellows_External[s] : Outport  Port=4
  LaneIdx_Fellows_External[] : Outport  Port=5
  wires:
  Const_LaneIdx_Fellows_External[]/1 -> LaneIdx_Fellows_External[]/1
  Const_tgap_Fellows_External[s]/1 -> tgap_Fellows_External[s]/1
  Const_v_Fellows_External[km|h]/1 -> v_Fellows_External[km|h]/1
  Const_d_Fellows_External[m]/1 -> d_Fellows_External[m]/1
  Const_s_Fellows_External[m]/1 -> s_Fellows_External[m]/1

== system ASM_Traffic_V2X_Complete_Model_2/MDL/Environment/Traffic/FellowMovement/LabelUserSignals ==
  UserSignals_In : Inport
  Bus Creator : BusCreator  Inputs=5
  UserSignals_ : Subsystem
  UserSignals : Outport
  wires:
  UserSignals_/5(User5[]) -> Bus Creator/5  "User5[]"
  UserSignals_/4(User4[]) -> Bus Creator/4  "User4[]"
  Bus Creator/1 -> UserSignals/1  "UserSignals"
  UserSignals_In/1 -> UserSignals_/1(UserSignals)
  UserSignals_/1(User1[]) -> Bus Creator/1  "User1[]"
  UserSignals_/2(User2[]) -> Bus Creator/2  "User2[]"
  UserSignals_/3(User3[]) -> Bus Creator/3  "User3[]"

== system ASM_Traffic_V2X_Complete_Model_2/MDL/Environment/Traffic/FellowMovement/LabelUserSignals_Fellows ==
  UserSignals_In : Inport
  Bus Creator : BusCreator  Inputs=15
  Selector : Selector  InputPortWidth=MDL.Traffic.MaxNumFellows.v*2  IndexOptions=Index vector (dialog)  Indices=[1:30]  OutputSizes=1
  UserSignals_ : Subsystem
  UserSignals_Fellows : Outport
  wires:
  Selector/1 -> UserSignals_/1(UserSignals)
  UserSignals_/4(UserSignals_Fellow4[]) -> Bus Creator/4  "UserSignals_Fellow4[]"
  UserSignals_/3(UserSignals_Fellow3[]) -> Bus Creator/3  "UserSignals_Fellow3[]"
  UserSignals_/2(UserSignals_Fellow2[]) -> Bus Creator/2  "UserSignals_Fellow2[]"
  UserSignals_/5(UserSignals_Fellow5[]) -> Bus Creator/5  "UserSignals_Fellow5[]"
  UserSignals_/6(UserSignals_Fellow6[]) -> Bus Creator/6  "UserSignals_Fellow6[]"
  UserSignals_/7(UserSignals_Fellow7[]) -> Bus Creator/7  "UserSignals_Fellow7[]"
  UserSignals_/14(UserSignals_Fellow14[]) -> Bus Creator/14  "UserSignals_Fellow14[]"
  UserSignals_/15(UserSignals_Fellow15[]) -> Bus Creator/15  "UserSignals_Fellow15[]"
  UserSignals_/13(UserSignals_Fellow13[]) -> Bus Creator/13  "UserSignals_Fellow13[]"
  UserSignals_/8(UserSignals_Fellow8[]) -> Bus Creator/8  "UserSignals_Fellow8[]"
  UserSignals_/9(UserSignals_Fellow9[]) -> Bus Creator/9  "UserSignals_Fellow9[]"
  UserSignals_/12(UserSignals_Fellow12[]) -> Bus Creator/12  "UserSignals_Fellow12[]"
  UserSignals_/10(UserSignals_Fellow10[]) -> Bus Creator/10  "UserSignals_Fellow10[]"
  UserSignals_/11(UserSignals_Fellow11[]) -> Bus Creator/11  "UserSignals_Fellow11[]"
  UserSignals_/1(UserSignals_Fellow1[]) -> Bus Creator/1  "UserSignals_Fellow1[]"
  UserSignals_In/1 -> Selector/1
  Bus Creator/1 -> UserSignals_Fellows/1  "UserSignals_Fellows"

== system ASM_Traffic_V2X_Complete_Model_2/MDL/Environment/Traffic/FellowMovement/Maneuver_Status_Handling ==
  ManeuverState[] : Inport
  Constant1 : Constant  Value=3
  Constant2 : Constant  Value=2
  Constant3 : Constant  Value=5
  Constant4 : Constant  Value=5
  Constant5 : Constant
  Constant6 : Constant  Value=0
  Constant7 : Constant  Value=2
  Constant8 : Constant  Value=0
  Logical Operator : Logic  AllPortsSameDT=off
  Logical Operator1 : Logic  AllPortsSameDT=off
  Memory : Memory
  Relational Operator : RelationalOperator  Operator===  RndMeth=Nearest  InputSameDT=on
  Relational Operator1 : RelationalOperator  Operator===  RndMeth=Nearest  InputSameDT=on
  Relational Operator2 : RelationalOperator  Operator===  RndMeth=Nearest  InputSameDT=on
  Relational Operator3 : RelationalOperator  Operator=~=  RndMeth=Nearest  InputSameDT=on
  Start : MultiPortSwitch  DataPortOrder=Zero-based contiguous  Inputs=2  zeroidx=on  SaturateOnIntegerOverflow=on
  "Stop " : MultiPortSwitch  DataPortOrder=Zero-based contiguous  Inputs=2  zeroidx=on  SaturateOnIntegerOverflow=on
  Sum1 : Sum  Inputs=|++  SaturateOnIntegerOverflow=on
  Traffic_Ctrl : Outport
  wires:
  Sum1/1 -> Traffic_Ctrl/1  "handling"
  ManeuverState[]/1 -> Relational Operator2/1, Relational Operator/1, Memory/1  "status"
  "Stop "/1 -> Sum1/2  "stop"
  Constant7/1 -> "Stop "/3
  Constant8/1 -> "Stop "/2
  Logical Operator1/1 -> "Stop "/1  "stop"
  Start/1 -> Sum1/1  "start"
  Constant5/1 -> Start/3
  Constant6/1 -> Start/2
  Logical Operator/1 -> Start/1
  Relational Operator3/1 -> Logical Operator1/2
  Relational Operator2/1 -> Logical Operator1/1
  Constant4/1 -> Relational Operator3/2
  Constant3/1 -> Relational Operator2/2
  Relational Operator1/1 -> Logical Operator/2
  Relational Operator/1 -> Logical Operator/1
  Constant2/1 -> Relational Operator1/2
  Constant1/1 -> Relational Operator/2
  Memory/1 -> Relational Operator3/1, Relational Operator1/1

== system ASM_Traffic_V2X_Complete_Model_2/MDL/Environment/Traffic/FellowMovement/SegmentEnd_External ==
  Const_SegmentEnd_External1[0|1] : Constant  Value=0
  Const_SegmentEnd_External2[0|1] : Constant  Value=0
  Const_SegmentEnd_External3[0|1] : Constant  Value=0
  Mux3 : Mux  Inputs=3
  SegmentEnd_External[0|1] : Outport
  wires:
  Mux3/1 -> SegmentEnd_External[0|1]/1
  Const_SegmentEnd_External1[0|1]/1 -> Mux3/1
  Const_SegmentEnd_External2[0|1]/1 -> Mux3/2
  Const_SegmentEnd_External3[0|1]/1 -> Mux3/3

== system ASM_Traffic_V2X_Complete_Model_2/MDL/Environment/Traffic/FellowMovement/Subsystem ==
  v_x_Vehicle[km|h] : Inport
  v_y_Vehicle[km|h] : Inport  Port=2
  Add : Sum
  Math Function : Math  Operator=square  OutputSignalType=real  SaturateOnIntegerOverflow=on
  Math Function1 : Math  Operator=square  OutputSignalType=real  SaturateOnIntegerOverflow=on
  Product : Product
  Sign : Signum
  Sqrt : Sqrt  SaturateOnIntegerOverflow=on
  v_Vehicle[km|h] : Outport
  wires:
  Product/1 -> v_Vehicle[km|h]/1
  Sqrt/1 -> Product/2
  Sign/1 -> Product/1
  v_x_Vehicle[km|h]/1 -> Math Function/1, Sign/1
  Add/1 -> Sqrt/1
  Math Function1/1 -> Add/2
  Math Function/1 -> Add/1
  v_y_Vehicle[km|h]/1 -> Math Function1/1

== system ASM_Traffic_V2X_Complete_Model_2/MDL/Environment/Traffic/FellowMovement/Sw_SpeedLimit_Enable ==
  SpeedLimit_In : Inport
  Multiport Switch : MultiPortSwitch  DataPortOrder=Zero-based contiguous  Inputs=2  DiagnosticForDefault=Warning  zeroidx=on
  SpeedLimit_Off[km|h] : Constant  Value=1000.0
  SpeedLimit_RateLimiter : Subsystem
  Sw_SpeedLimit_Enable[0Off|1On] : Constant  Value=[ones(1,MDL.Traffic.MaxNumFellows.v)]  OutDataTypeStr=uint8
  SpeedLimit_Out : Outport
  wires:
  SpeedLimit_In/1 -> SpeedLimit_RateLimiter/1(In)
  SpeedLimit_RateLimiter/1(Out) -> Multiport Switch/3
  SpeedLimit_Off[km|h]/1 -> Multiport Switch/2
  Multiport Switch/1 -> SpeedLimit_Out/1
  Sw_SpeedLimit_Enable[0Off|1On]/1 -> Multiport Switch/1

== system ASM_Traffic_V2X_Complete_Model_2/MDL/Environment/Traffic/ObjectParameters/ASMSignalCollector ==
  Bus Creator1 : BusCreator  Inputs=3
  tag scope: ASMBUS_Environment_Traffic_ObjectParameters=global
  wires:
  [ASMBUS_Environment_Traffic_DiscreteObjects] -> Bus Creator1/3
  Bus Creator1/1 -> [ASMBUS_Environment_Traffic_ObjectParameters]  "ObjectParameters"
  [ASMBUS_Environment_Traffic_FellowParameters] -> Bus Creator1/1
  [ASMBUS_Environment_Traffic_TrafficObjects] -> Bus Creator1/2

== system ASM_Traffic_V2X_Complete_Model_2/MDL/Environment/Traffic/ObjectParameters/Object_Reload_Trigger ==
  RoadCtrl[] : Inport
  Constant1 : Constant
  Constant2 : Constant
  Constant5 : Constant
  Constant6 : Constant  Value=0
  Logical Operator : Logic  AllPortsSameDT=off
  Memory : Memory
  Relational Operator : RelationalOperator  Operator===  RndMeth=Nearest  InputSameDT=on
  Relational Operator1 : RelationalOperator  Operator=~=  RndMeth=Nearest  InputSameDT=on
  Start : MultiPortSwitch  DataPortOrder=Zero-based contiguous  Inputs=2  zeroidx=on  SaturateOnIntegerOverflow=on
  Ctrl : Outport
  wires:
  Memory/1 -> Relational Operator1/1
  Constant1/1 -> Relational Operator/2
  Constant2/1 -> Relational Operator1/2
  Relational Operator/1 -> Logical Operator/1
  Relational Operator1/1 -> Logical Operator/2
  Logical Operator/1 -> Start/1
  Constant6/1 -> Start/2
  Constant5/1 -> Start/3
  Start/1 -> Ctrl/1  "start"
  RoadCtrl[]/1 -> Relational Operator/1, Memory/1  "status"

== system ASM_Traffic_V2X_Complete_Model_2/MDL/Environment/Traffic/Sensors/ASMSignalCollector ==
  Bus Creator1 : BusCreator  Inputs=7
  tag scope: ASMBUS_Environment_Traffic_Sensors=global
  wires:
  [ASMBUS_Environment_Traffic_Sensors_Collision_Sensor] -> Bus Creator1/6
  [ASMBUS_Environment_Traffic_Sensors_Line_Sensor] -> Bus Creator1/5
  [ASMBUS_Environment_Traffic_Sensors_Common] -> Bus Creator1/7
  [ASMBUS_Environment_Traffic_Sensors_Object_Sensor_2D] -> Bus Creator1/2
  [ASMBUS_Environment_Traffic_Sensors_Custom_Sensor] -> Bus Creator1/4
  Bus Creator1/1 -> [ASMBUS_Environment_Traffic_Sensors]  "Sensors"
  [ASMBUS_Environment_Trafffic_Sensors_Object_Sensor_3D] -> Bus Creator1/1
  [ASMBUS_Environment_Traffic_Sensors_Traffic_Sign_Sensor_dyn] -> Bus Creator1/3

== system ASM_Traffic_V2X_Complete_Model_2/MDL/Environment/Traffic/Sensors/Collision_Sensor ==
  Enable[0Off|1On] : Inport
  Fellows_Signals : Inport  Port=2
  VehicleDynamics_Signals : Inport  Port=3
  Objects_Signals : Inport  Port=4
  Road_Signals : Inport  Port=5
  Maneuver_Signals : Inport  Port=6
  ASMSignalCollector : Subsystem
  Bus Selector : BusSelector  OutputSignals=Flag_FellowUsed[0|1],Pos_Fellows_MainPnt_CoorSys_E[x;y;z][m],Angle_Fellows[x;y;z][deg],v_Fellows[x;y;z][km|h],w_Fellows[x;y;z][deg|s]
  Bus Selector1 : BusSelector  OutputSignals=VehicleMovement.Positions.Pos_Vehicle_CoorSys_E[x;y;z][m].Pos_Vehicle_CoorSys_E[x;y;z][m],VehicleMovement.Positions.Angle_Vehicle_CoorSys_E[x;y;z][deg].Angle_Vehicle_CoorSys_E[x;y;z][deg],VehicleMovement.Velocities.v_x_Vehicle[km|h],VehicleMovement.Velocities.v_y_Vehicle[km|h],VehicleMovement.Velocities.YawRate_Vehicle[deg|s]
  Bus Selector2 : BusSelector  OutputSignals=TrafficObject_Type_Fellows[],TrafficObject_Type_Data[],DiscreteObject_Data[]
  Bus Selector3 : BusSelector  OutputSignals=TrafficObject_Data[]
  Bus Selector4 : BusSelector  OutputSignals=TrafficObject_Type_CollisionObj[],Pos_x_CollisionObj_Custom_RefPnt[m],Pos_y_CollisionObj_Custom_RefPnt[m]
  Bus Selector5 : BusSelector  OutputSignals=Info.ManeuverTime[s],Parameters.Object_Type_ID[]
  COLLISION_SENSOR : ASM_Traffic_lib/Sensors/Collision_Sensor/COLLISION_SENSOR  Tag=ASM_SUBCOMPONENT  Sw_Sensor_Enable=MDL.Traffic.Sensors.CollisionSensor.Sw_Sensor_Enable  Sw_Detection_Mode=MDL.Traffic.Sensors.CollisionSensor.Sw_Detection_Mode  Const_Collisions_OutputDimension=MDL.Traffic.Sensors.CollisionSensor.Const_Sensor_Output_Dimension  ASMProperties=struct('Name','COLLISION_SENSOR','Version','1.0','Library','ASM_Traffic_lib')  ASMInstanceName=collision_sensor  ASMInstanceID=1
  Constant : Constant  Value=0
  Demux : Demux  Outputs=3
  Enable_Collision_Sensor : Subsystem
  Mux : Mux  Inputs=3
  Mux1 : Mux  Inputs=2
  Terminator : Terminator
  Terminator2 : Terminator
  Sensor_Signals : Outport
  tag scope: ASMBUS_Traf_Sensors_Collision_Sensor_1=global
  wires:
  Bus Selector4/3 -> Mux1/2  "<Pos_y_CollisionObj_Custom_RefPnt[m]>"
  Bus Selector4/2 -> Mux1/1  "<Pos_x_CollisionObj_Custom_RefPnt[m]>"
  [TAG_CollisionSensor_Parameters] -> Bus Selector4/1
  Bus Selector/4 -> COLLISION_SENSOR/11  "<v_Fellows[x;y;z][km|h]>"
  Bus Selector/5 -> Demux/1  "<w_Fellows[x;y;z][deg|s]>"
  Demux/3 -> COLLISION_SENSOR/12
  Demux/1 -> Terminator/1
  Demux/2 -> Terminator2/1
  Constant/1 -> Mux/3
  Bus Selector5/1 -> COLLISION_SENSOR/6  "<ManeuverTime[s]>"
  Bus Selector5/2 -> COLLISION_SENSOR/7  "<Object_Type_ID[]>"
  Maneuver_Signals/1 -> Bus Selector5/1
  Mux/1 -> COLLISION_SENSOR/4
  COLLISION_SENSOR/1 -> [ASMBUS_Traf_Sensors_Collision_Sensor_1]
  COLLISION_SENSOR/2 -> Sensor_Signals/1
  Bus Selector3/1 -> COLLISION_SENSOR/18  "<TrafficObject_Data[]>"
  Bus Selector2/3 -> COLLISION_SENSOR/17  "<DiscreteObject_Data[]>"
  Bus Selector2/2 -> COLLISION_SENSOR/16  "<TrafficObject_Type_Data[]>"
  Bus Selector2/1 -> COLLISION_SENSOR/15  "<TrafficObject_Type_Fellows[]>"
  Mux1/1 -> COLLISION_SENSOR/14
  Bus Selector4/1 -> COLLISION_SENSOR/13  "<TrafficObject_Type_CollisionObj[]>"
  Bus Selector/1 -> COLLISION_SENSOR/8  "<Flag_FellowUsed[0|1]>"
  Bus Selector1/5 -> COLLISION_SENSOR/5  "<YawRate_Vehicle[deg|s]>"
  Bus Selector1/4 -> Mux/2  "<v_y_Vehicle[km|h]>"
  Bus Selector1/3 -> Mux/1  "<v_x_Vehicle[km|h]>"
  Bus Selector1/2 -> COLLISION_SENSOR/3  "<Angle_Vehicle_CoorSys_E[x;y;z][deg]>"
  Bus Selector1/1 -> COLLISION_SENSOR/2  "<Pos_Vehicle_CoorSys_E[x;y;z][m]>"
  Enable_Collision_Sensor/1(Enable_Out[0Off|1On]) -> COLLISION_SENSOR/1
  Enable[0Off|1On]/1 -> Enable_Collision_Sensor/1(Enable_In[0Off|1On])
  VehicleDynamics_Signals/1 -> Bus Selector1/1
  Fellows_Signals/1 -> Bus Selector/1
  Bus Selector/2 -> COLLISION_SENSOR/9  "<Pos_Fellows_MainPnt_CoorSys_E[x;y;z][m]>"
  Bus Selector/3 -> COLLISION_SENSOR/10  "<Angle_Fellows[x;y;z][deg]>"
  Road_Signals/1 -> Bus Selector3/1
  Objects_Signals/1 -> Bus Selector2/1
